simulink model "lwdf_butter5_faulty"  (R2014b)
settings: Solver=ode45  StartTime=0.0  StopTime=10.0  RelTol=1e-3
undefined symbols (not defined in the file): lwdf_adaptors, type1
settings Model: Creator=ravoson  LastModifiedBy=ravoson

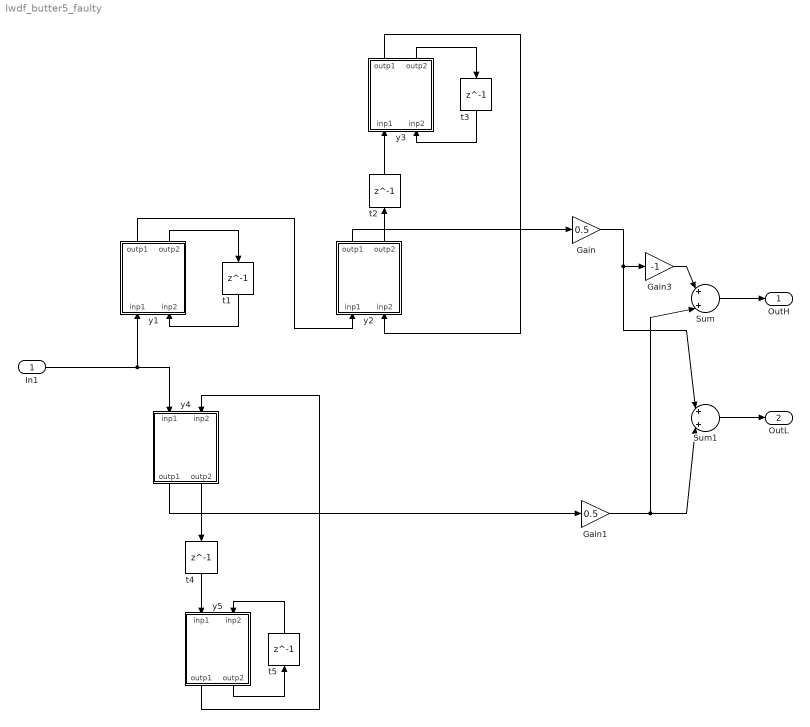
== system lwdf_butter5_faulty ==
  In1 : Inport
  Gain : Gain  Gain=0.5
  Gain1 : Gain  Gain=0.5
  Gain3 : Gain  Gain=-1
  Sum : Sum  Inputs=|+|+|
  Sum1 : Sum  Inputs=|+|+|
  t{1..5} (5 alike) : Delay  DelayLength=1  InitialCondition=0
  y1 : Subsystem
  y2 : Subsystem
  y3 : Subsystem  AncestorBlock=lwdf_adaptors/type1
  y4 : Subsystem
  y5 : Subsystem
  OutH : Outport
  OutL : Outport  Port=2
  wires:
  y1/2(outp2) -> t1/1
  t1/1 -> y1/2(inp2)
  In1/1 -> y4/1(inp1), y1/1(inp1)
  y1/1(outp1) -> y2/1(inp1)
  y2/1(outp1) -> Gain/1
  y2/2(outp2) -> t2/1
  t2/1 -> y3/1(inp1)
  t3/1 -> y3/2(inp2)
  y3/2(outp2) -> t3/1
  y3/1(outp1) -> y2/2(inp2)
  y4/2(outp2) -> t4/1
  t4/1 -> y5/1(inp1)
  t5/1 -> y5/2(inp2)
  y5/2(outp2) -> t5/1
  y4/1(outp1) -> Gain1/1
  y5/1(outp1) -> y4/2(inp2)
  Gain3/1 -> Sum/1
  Gain/1 -> Sum1/1, Gain3/1
  Sum1/1 -> OutL/1
  Sum/1 -> OutH/1
  Gain1/1 -> Sum1/2, Sum/2

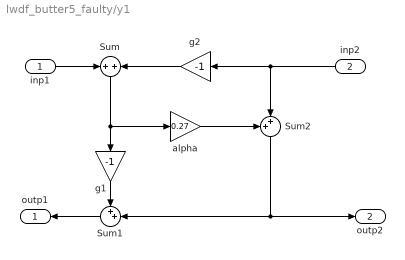
== system lwdf_butter5_faulty/y1 ==
  inp1 : Inport
  inp2 : Inport  Port=2
  Sum : Sum  Inputs=+|+
  Sum1 : Sum  Inputs=++|
  Sum2 : Sum  Inputs=++|
  alpha : Gain  Gain=0.27
  g1 : Gain  Gain=-1
  g2 : Gain  Gain=-1
  outp1 : Outport
  outp2 : Outport  Port=2
  wires:
  g2/1 -> Sum/2
  Sum1/1 -> outp1/1
  inp2/1 -> g2/1, Sum2/2
  Sum2/1 -> Sum1/2, outp2/1
  inp1/1 -> Sum/1
  g1/1 -> Sum1/1
  Sum/1 -> g1/1, alpha/1
  alpha/1 -> Sum2/1

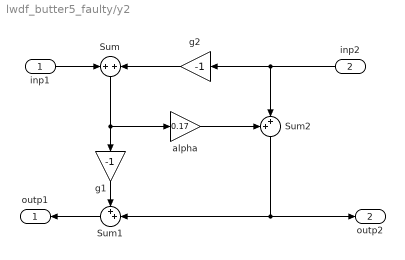
== system lwdf_butter5_faulty/y2 ==
  inp1 : Inport
  inp2 : Inport  Port=2
  Sum : Sum  Inputs=+|+
  Sum1 : Sum  Inputs=++|
  Sum2 : Sum  Inputs=++|
  alpha : Gain  Gain=0.17
  g1 : Gain  Gain=-1
  g2 : Gain  Gain=-1
  outp1 : Outport
  outp2 : Outport  Port=2
  wires:
  g2/1 -> Sum/2
  Sum1/1 -> outp1/1
  inp2/1 -> g2/1, Sum2/2
  Sum2/1 -> Sum1/2, outp2/1
  inp1/1 -> Sum/1
  g1/1 -> Sum1/1
  Sum/1 -> g1/1, alpha/1
  alpha/1 -> Sum2/1

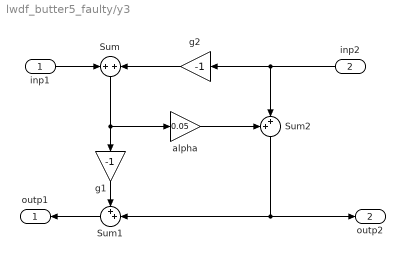
== system lwdf_butter5_faulty/y3 ==
  inp1 : Inport
  inp2 : Inport  Port=2
  Sum : Sum  Inputs=+|+
  Sum1 : Sum  Inputs=++|
  Sum2 : Sum  Inputs=++|
  alpha : Gain  Gain=0.05
  g1 : Gain  Gain=-1
  g2 : Gain  Gain=-1
  outp1 : Outport
  outp2 : Outport  Port=2
  wires:
  g2/1 -> Sum/2
  Sum1/1 -> outp1/1
  inp2/1 -> g2/1, Sum2/2
  Sum2/1 -> Sum1/2, outp2/1
  inp1/1 -> Sum/1
  g1/1 -> Sum1/1
  Sum/1 -> g1/1, alpha/1
  alpha/1 -> Sum2/1

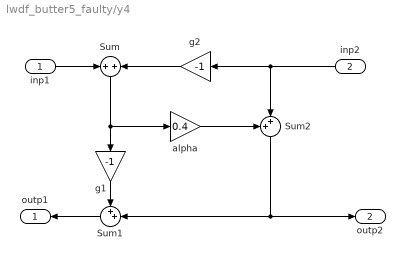
== system lwdf_butter5_faulty/y4 ==
  inp1 : Inport
  inp2 : Inport  Port=2
  Sum : Sum  Inputs=+|+
  Sum1 : Sum  Inputs=++|
  Sum2 : Sum  Inputs=++|
  alpha : Gain  Gain=0.4
  g1 : Gain  Gain=-1
  g2 : Gain  Gain=-1
  outp1 : Outport
  outp2 : Outport  Port=2
  wires:
  g2/1 -> Sum/2
  Sum1/1 -> outp1/1
  inp2/1 -> g2/1, Sum2/2
  Sum2/1 -> Sum1/2, outp2/1
  inp1/1 -> Sum/1
  g1/1 -> Sum1/1
  Sum/1 -> g1/1, alpha/1
  alpha/1 -> Sum2/1

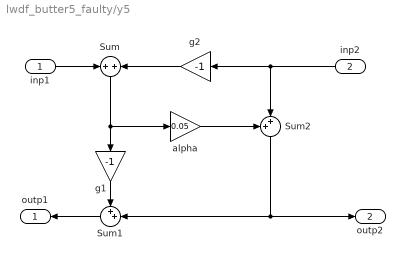
== system lwdf_butter5_faulty/y5 ==
  inp1 : Inport
  inp2 : Inport  Port=2
  Sum : Sum  Inputs=+|+
  Sum1 : Sum  Inputs=++|
  Sum2 : Sum  Inputs=++|
  alpha : Gain  Gain=0.05
  g1 : Gain  Gain=-1
  g2 : Gain  Gain=-1
  outp1 : Outport
  outp2 : Outport  Port=2
  wires:
  g2/1 -> Sum/2
  Sum1/1 -> outp1/1
  inp2/1 -> g2/1, Sum2/2
  Sum2/1 -> Sum1/2, outp2/1
  inp1/1 -> Sum/1
  g1/1 -> Sum1/1
  Sum/1 -> g1/1, alpha/1
  alpha/1 -> Sum2/1
